simulink model "MASTER"  (R2024b)
settings: Solver=FixedStepAuto  StartTime=0.0  StopTime=10.0  RelTol=1e-3  EnableMultiTasking=on
libraries: simulink x1
settings Model: DataDictionary=Master_Dictionary.sldd  EnableAccessToBaseWorkspace=off  TickDuration=2.0E-08  Creator=torni  LastModifiedBy=Will
settings OptimizationCC: DefaultParameterBehavior=Inlined  EnhancedBackFolding=on  PassReuseOutputArgsAs=Individual arguments  ZeroExternalMemoryAtStartup=off  ZeroInternalMemoryAtStartup=off  MaxStackSize=8192  OptimizeBlockOrder=speed  DifferentSizesBufferReuse=on  OptimizationCustomize=off  EfficientTunableParamExpr=on
settings DebuggingCC: ParameterTunabilityLossMsg=error
settings HardwareCC: ProdBitPerPointer=32  ProdBitPerSizeT=32  ProdBitPerPtrDiffT=32  ProdLargestAtomicInteger=Long  ProdLargestAtomicFloat=Double  ProdWordSize=32  ProdLongLongMode=on  ProdHWDeviceType=ARM Compatible->ARM Cortex-M
settings SFSimCC: MATLABDynamicMemAlloc=off
settings RTWCC: Description=Embedded Coder  SystemTargetFile=ert.tlc  HardwareBoard=STM32H7xx Based (Single-core)  TemplateMakefile=ert_default_tmf  Toolchain=GNU Tools for ARM Embedded Processors
settings CodeAppCC: ForceParamTrailComments=on  IgnoreCustomStorageClasses=off  OperatorAnnotations=on  SimulinkDataObjDesc=on  SFDataObjDesc=on  InsertBlockDesc=on
settings ERTTargetCC: TargetLangStandard=C99 (ISO)  CodeReplacementLibrary=ARM Cortex-M  ExtModeTransport=3  ExtModeStaticAlloc=on  ExtModeStaticAllocSize=2048  ExtModeMexFile=ext_xcp  ExtModeIntrfLevel=Level2 - Open

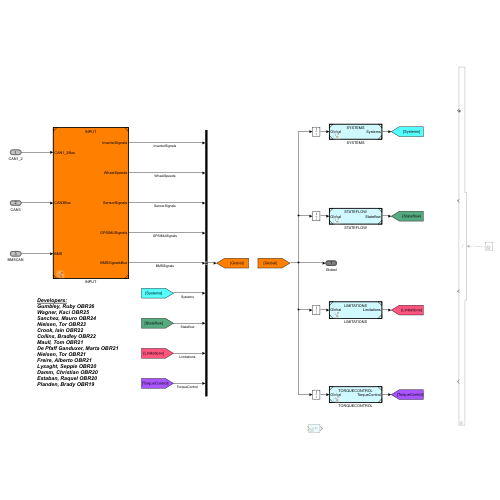
[thumbnail: Simulink's stored preview of the top-level diagram]
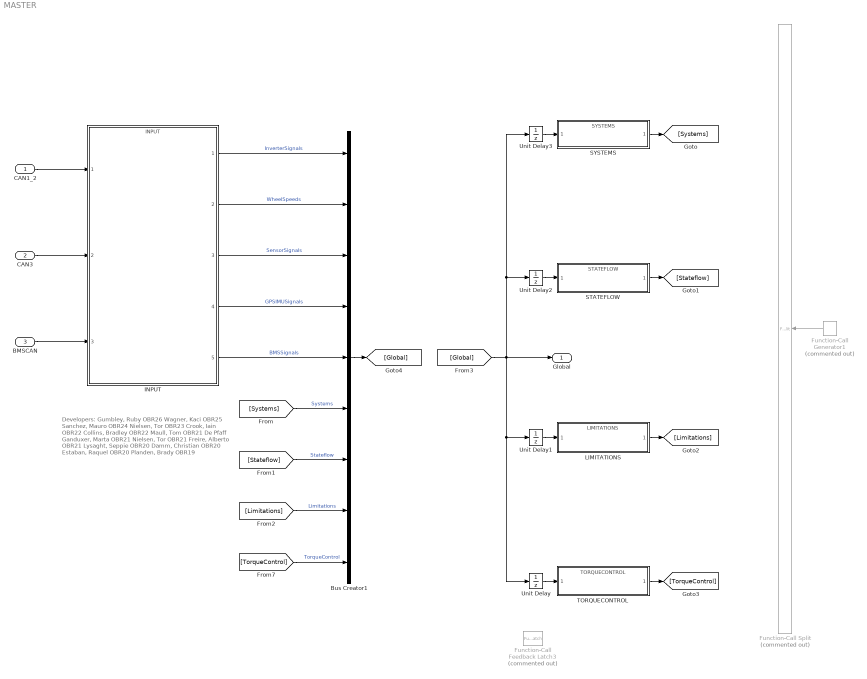
== system MASTER ==
  note: Developers:
      | Gumbley, Ruby OBR26
      | Wagner, Kaci OBR25
      | Sanchez, Mauro OBR24
      | Nielsen, Tor OBR23
      | Crook, Iain OBR22
      | Collins, Bradley OBR22
      | Maull, Tom OBR21
      | De Pfaff Ganduxer, Marta OBR21
      | Nielsen, Tor OBR21
      | Freire, Alberto OBR21
      | Lysaght, Seppie OBR20
      | Damm, Christian OBR20
      | Estaban, Raquel OBR20
      | Planden, Brady OBR19
  CAN1_2 : Inport  OutDataTypeStr=Bus: CAN1_2Bus
  CAN3 : Inport  Port=2  OutDataTypeStr=Bus: CAN3Bus
  BMSCAN : Inport  Port=3  OutDataTypeStr=Bus: BMS
  Bus Creator1 : BusCreator  Inputs=9  OutDataTypeStr=Bus: Global
  Function-Call Feedback Latch3 : FunctionCallFeedbackLatch  Commented=on
  Function-Call Generator1 : simulink/Ports & Subsystems/Function-Call Generator  Commented=on  sample_time=-1  numberOfIterations=1  DisallowWideOutput=off
  Function-Call Split : FunctionCallSplit  Commented=on  IconShape=distinctive  NumOutputPorts=4  OutputPortLayout=default
  INPUT : ModelReference  ModelNameDialog=INPUT  SimulationMode=Normal  ModelReferenceVersion=13.8
  LIMITATIONS : ModelReference  ModelNameDialog=LIMITATIONS  SimulationMode=Normal  ModelReferenceVersion=13.8
  STATEFLOW : ModelReference  ModelNameDialog=STATEFLOW  SimulationMode=Normal  ModelReferenceVersion=13.8
  SYSTEMS : ModelReference  ModelNameDialog=SYSTEMS  SimulationMode=Normal  ModelReferenceVersion=13.10
  TORQUECONTROL : ModelReference  ModelNameDialog=TORQUECONTROL  SimulationMode=Normal  ModelReferenceVersion=13.8
  Unit Delay{,1..3} (4 alike) : UnitDelay  SampleTime=-1  HasFrameUpgradeWarning=on
  Global : Outport  OutDataTypeStr=Bus: Global  VectorParamsAs1DForOutWhenUnconnected=off
  wires:
  INPUT/1 -> Bus Creator1/1  "InverterSignals"
  INPUT/2 -> Bus Creator1/2  "WheelSpeeds"
  INPUT/3 -> Bus Creator1/3  "SensorSignals"
  INPUT/4 -> Bus Creator1/4  "GPSIMUSignals"
  [Global] -> Unit Delay/1, Unit Delay1/1, Global/1, Unit Delay3/1, Unit Delay2/1
  SYSTEMS/1 -> [Systems]
  [Systems] -> Bus Creator1/6  "Systems"
  STATEFLOW/1 -> [Stateflow]
  [Stateflow] -> Bus Creator1/7  "Stateflow"
  LIMITATIONS/1 -> [Limitations]
  [Limitations] -> Bus Creator1/8  "Limitations"
  TORQUECONTROL/1 -> [TorqueControl]
  INPUT/5 -> Bus Creator1/5  "BMSSignals"
  [TorqueControl] -> Bus Creator1/9  "TorqueControl"
  Bus Creator1/1 -> [Global]
  Function-Call Generator1/1 -> Function-Call Split/1
  CAN1_2/1 -> INPUT/1
  CAN3/1 -> INPUT/2
  BMSCAN/1 -> INPUT/3
  Unit Delay/1 -> TORQUECONTROL/1
  Unit Delay1/1 -> LIMITATIONS/1
  Unit Delay2/1 -> STATEFLOW/1
  Unit Delay3/1 -> SYSTEMS/1
